simulink library "command_handler_lib"  (Simulink 8.2)
settings: Solver=ode1  StartTime=0.0  StopTime=Inf  FixedStep=0.001  RelTol=1e-3
PostLoadFcn:
  | , if any(exist('dsrtsu_mdlpostloadfcn', 'file') == [2, 3, 6]), try dsrtsu_mdlpostloadfcn('Execute', bdroot); catch fprintf('Error in PostLoadFcn (dsrtsu_mdlpostloadfcn) for model "%s":\n %s\n', bdroot, lasterr); end, end,
settings Model: DSRTSU_INTERNAL_RTI_VER=450  DSRTSU_INTERNAL_RTI_TYPE=rti1401  DSRTSU_INTERNAL_RTIFPGA=40  Creator=rushk1  LastModifiedBy=rushk1

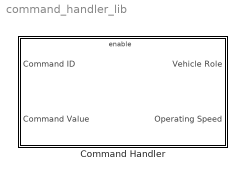
== system command_handler_lib ==
  Command Handler : Subsystem

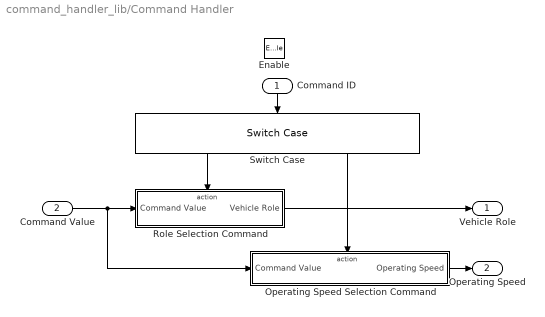
== system command_handler_lib/Command Handler ==
  Command ID : Inport
  Command Value : Inport  Port=2
  Enable : EnablePort
  Operating Speed Selection Command : Subsystem  TreatAsAtomicUnit=on
  Role Selection Command : Subsystem  TreatAsAtomicUnit=on
  Switch Case : SwitchCase  CaseConditions={129, 130}  ShowDefaultCase=off
  Vehicle Role : Outport
  Operating Speed : Outport  Port=2
  wires:
  Role Selection Command/1(Vehicle Role) -> Vehicle Role/1
  Operating Speed Selection Command/1(Operating Speed) -> Operating Speed/1
  Command Value/1 -> Role Selection Command/1(Command Value), Operating Speed Selection Command/1(Command Value)
  Switch Case/2 -> Operating Speed Selection Command/Action
  Switch Case/1 -> Role Selection Command/Action
  Command ID/1 -> Switch Case/1

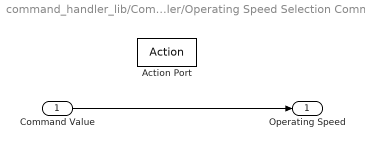
== system command_handler_lib/Command Handler/Operating Speed Selection Command ==
  Command Value : Inport
  Action Port : ActionPort
  Operating Speed : Outport
  wires:
  Command Value/1 -> Operating Speed/1

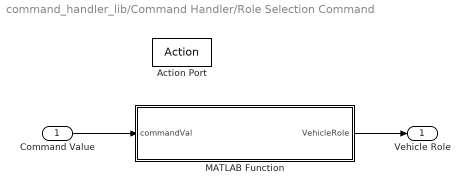
== system command_handler_lib/Command Handler/Role Selection Command ==
  Command Value : Inport
  Action Port : ActionPort
  MATLAB Function : MATLAB Function  TreatAsAtomicUnit=on
  Vehicle Role : Outport
  wires:
  Command Value/1 -> MATLAB Function/1(commandVal)
  MATLAB Function/1(VehicleRole) -> Vehicle Role/1

== matlab function Command Handler/Role Selection Command/MATLAB Function ==
  data: commandVal input double; VehicleRole output double
function VehicleRole = convertVehicleRole(commandVal)
%#codegen
VehicleRole = VehicleRoleEnum(commandVal);
